simulink model "playing"  (R2019a)
settings: Solver=FixedStepAuto  StartTime=0.0  StopTime=100.0  RelTol=1e-3
libraries: simulink x1
settings Model: Creator=celit  LastModifiedBy=celit

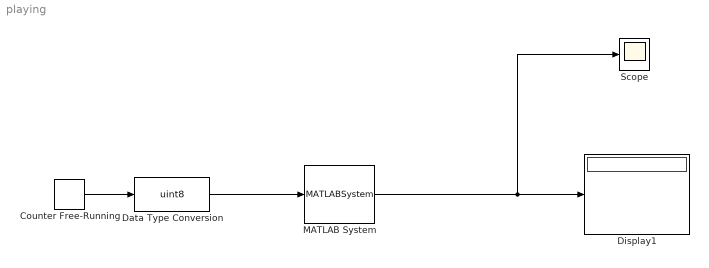
== system playing ==
  Counter Free-Running : simulink/Sources/Counter Free-Running  NumBits=16  tsamp=.1
  Data Type Conversion : DataTypeConversion  OutDataTypeStr=uint8
  Display1 : Display
  MATLAB System : MATLABSystem  System=MonoDrive  SimulateUsing=Interpreted execution
      mask Type: MonoDrive
      mask Display:
      | disp('MonoDrive');
      | port_label('input',1,'u');
      | port_label('output',1,'y');
  Scope : Scope
  wires:
  Counter Free-Running/1 -> Data Type Conversion/1
  MATLAB System/1 -> Scope/1, Display1/1
  Data Type Conversion/1 -> MATLAB System/1
